simulink model "ModelAudDetect"  (R2024b)
settings: Solver=VariableStepAuto  StartTime=0.0  StopTime=10.0  RelTol=1e-3
undefined symbols (not defined in the file or in its folder): Radix
libraries: audiosources x1, dspxfrm3 x1, dspsigops x1
settings Model: Creator=Manav  LastModifiedBy=Manav

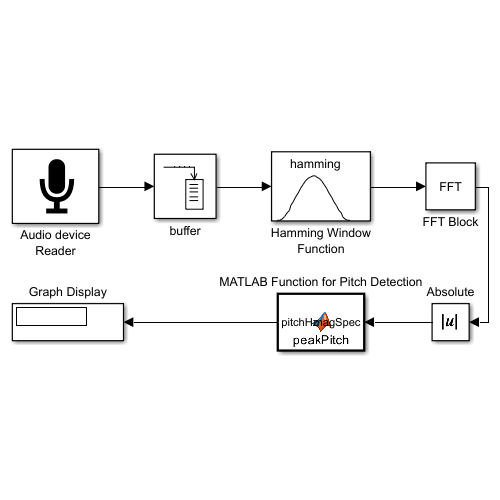
[thumbnail: Simulink's stored preview of the top-level diagram]
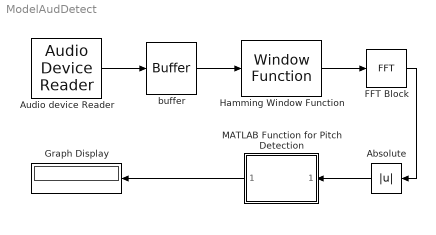
== system ModelAudDetect ==
  Absolute : Abs  SaturateOnIntegerOverflow=off
  Audio device Reader : audiosources/Audio Device Reader  Driver=DirectSound  Device=Default  SampleRate=16000  NumChannels=1  SamplesPerFrame=2048  BitDepth=16-bit integer  NumBuffers=10  DefaultInputChannelMapping=on  InputChannelMapping=1:2  OutputNumOverrunSamples=off  OutputDataType=double  DriverIdx=1  DeviceWarnFlag=''
  FFT Block : dspxfrm3/FFT  FFTImplementation=Radix-2  CompMethod=Table lookup  TableOpt=NEW  TableOptActive=Speed  BitRevOrder=off  Normalize=off  InheritFFTLength=on  FFTLength=64  WrapInput=on  roundingMode=Ceiling  overflowMode=off  firstCoeffDataTypeStr=Inherit: Same word length as input  firstCoeffLastDataTypeStr=Inherit: Same word length as input  outputMin=[]  outputMax=[]
  Graph Display : Display
  Hamming Window Function : dspsigops/Window Function  winmode=Apply window to input  wintype=Hamming  sampmode=Continuous  samptime=1  N=64  Rs=50  beta=10  winsamp=Symmetric  UserWindow=hamming  OptParams=off  UserParams={'symmetric'}  dataType=double  isSigned=on  wordLen=16  udDataType=sfix(16)  fracBitsMode=Best precision  numFracBits=15  roundingMode=Floor  overflowMode=off  numSidelobes=4  sidelobeLevel=-30
  MATLAB Function for Pitch Detection : MATLAB Function  TreatAsAtomicUnit=on
  buffer : Buffer  N=2048  OutputFrames=off
  wires:
  FFT Block/1 -> Absolute/1
  Hamming Window Function/1 -> FFT Block/1
  buffer/1 -> Hamming Window Function/1
  Absolute/1 -> MATLAB Function for Pitch Detection/1(magSpec)
  Audio device Reader/1 -> buffer/1
  MATLAB Function for Pitch Detection/1(pitchHz) -> Graph Display/1

== matlab function ModelAudDetect/MATLAB Function for Pitch Detection ==
  data: magSpec input; pitchHz output
function pitchHz = peakPitch(magSpec)

fs = 16000;     
N  = 2048;      
fmin = 50;
fmax = 500;

halfN = N/2;
spec = magSpec(1:halfN);

kmin = ceil(fmin * N / fs);
kmax = floor(fmax * N / fs);

kmin = max(kmin,1);
kmax = min(kmax,halfN);

[~, idx] = max(spec(kmin:kmax));
k = kmin + idx - 1;

pitchHz = (k * fs) / N;
end
